simulink model "ps3"  (R2020b)
settings: Solver=VariableStepAuto  StartTime=0.0  StopTime=10.0  RelTol=1e-3
settings Model: Creator=prana  LastModifiedBy=prana

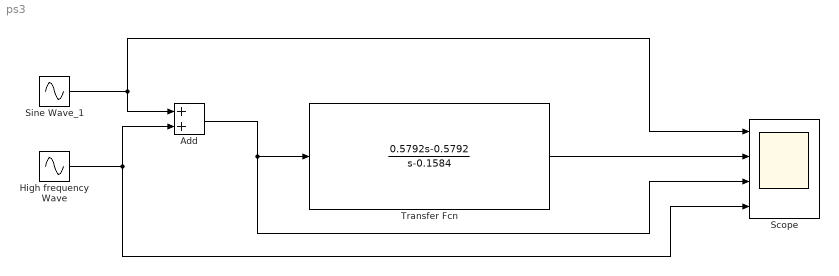
== system ps3 ==
  Add : Sum
  High frequency Wave : Sin  SampleTime=0
  Scope : Scope  NumInputPorts=4
  Sine Wave_1 : Sin  SampleTime=0
  Transfer Fcn : TransferFcn  Numerator=[0.5792 -0.5792]  Denominator=[1 -0.1584]
  wires:
  Transfer Fcn/1 -> Scope/2
  Sine Wave_1/1 -> Add/1, Scope/1
  High frequency Wave/1 -> Scope/4, Add/2
  Add/1 -> Scope/3, Transfer Fcn/1
